simulink model "lawsdigital11"  (R2022b)
settings: Solver=VariableStepAuto  StartTime=0.0  StopTime=10.0  RelTol=1e-3
settings Model: Creator=vijit  LastModifiedBy=vijit

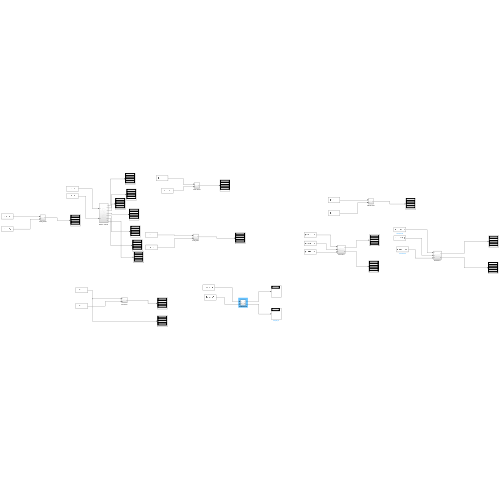
[thumbnail: Simulink's stored preview of the top-level diagram]
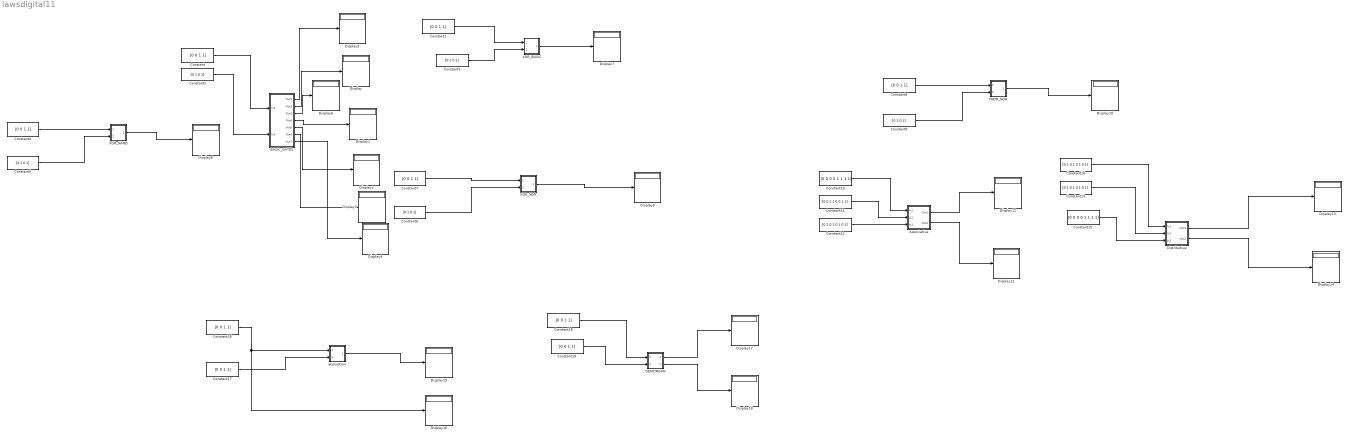
== system lawsdigital11 ==
  Associative : Subsystem
  BASIC_GATES : Subsystem
  Constant{,2,4,7..8,16..19} (9 alike) : Constant  Value=[0 0 1 1]
  Constant{1,3,5..6,9} (5 alike) : Constant  Value=[0 1 0 1]
  Constant10 : Constant  Value=[0 0 0 0 1 1 1 1]
  Constant11 : Constant  Value=[0 0 1 1 0 0 1 1]
  Constant12 : Constant  Value=[0 1 0 1 0 1 0 1]
  Constant13 : Constant  Value=[0 1 0 1 0 1 0 1]
  Constant14 : Constant  Value=[0 1 0 1 0 1 0 1]
  Constant15 : Constant  Value=[0 0 0 0 1 1 1 1]
  DEMORGAN : Subsystem
  Display{,1..18} (19 alike) : Display
  Distributive : Subsystem
  XNOR_NOR : Subsystem
  XOR_BASIC : Subsystem
  XOR_NAND : Subsystem
  XOR_NOR : Subsystem
  absorption : Subsystem
  wires:
  Constant3/1 -> XOR_BASIC/2(In2)
  Constant2/1 -> XOR_BASIC/1(In1)
  XOR_BASIC/1(Out1) -> Display7/1
  Constant/1 -> BASIC_GATES/1(In1)
  Constant1/1 -> BASIC_GATES/2(In2)
  BASIC_GATES/1(Out1) -> Display5/1
  BASIC_GATES/2(Out2) -> Display/1
  BASIC_GATES/3(Out3) -> Display6/1
  BASIC_GATES/4(Out4) -> Display1/1
  BASIC_GATES/5(Out5) -> Display2/1
  BASIC_GATES/6(Out6) -> Display3/1
  BASIC_GATES/7(Out7) -> Display4/1
  Constant4/1 -> XOR_NAND/1(In1)
  Constant5/1 -> XOR_NAND/2(In2)
  XOR_NAND/1(Out1) -> Display8/1
  Constant7/1 -> XOR_NOR/1(In1)
  Constant6/1 -> XOR_NOR/2(In2)
  XOR_NOR/1(Out1) -> Display9/1
  Constant8/1 -> XNOR_NOR/1(In1)
  Constant9/1 -> XNOR_NOR/2(In2)
  XNOR_NOR/1(Out1) -> Display10/1
  Constant10/1 -> Associative/1(In1)
  Constant11/1 -> Associative/2(In2)
  Constant12/1 -> Associative/3(In3)
  Associative/1(Out1) -> Display11/1
  Associative/2(Out2) -> Display12/1
  Constant14/1 -> Distributive/1(In1)
  Constant13/1 -> Distributive/2(In2)
  Constant15/1 -> Distributive/3(In3)
  Distributive/1(Out1) -> Display13/1
  Distributive/2(Out2) -> Display14/1
  Constant16/1 -> absorption/1(In1), Display16/1
  Constant17/1 -> absorption/2(In2)
  absorption/1(Out1) -> Display15/1
  Constant18/1 -> DEMORGAN/1(In1)
  Constant19/1 -> DEMORGAN/2(In2)
  DEMORGAN/1(Out1) -> Display17/1
  DEMORGAN/2(Out2) -> Display18/1

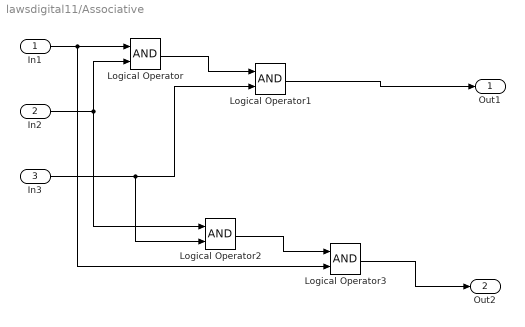
== system lawsdigital11/Associative ==
  In1 : Inport
  In2 : Inport  Port=2
  In3 : Inport  Port=3
  Logical Operator{,1..3} (4 alike) : Logic  AllPortsSameDT=off  OutDataTypeStr=boolean
  Out1 : Outport
  Out2 : Outport  Port=2
  wires:
  In3/1 -> Logical Operator2/2, Logical Operator1/2
  Logical Operator2/1 -> Logical Operator3/1
  In1/1 -> Logical Operator3/2, Logical Operator/1
  Logical Operator3/1 -> Out2/1
  In2/1 -> Logical Operator/2, Logical Operator2/1
  Logical Operator/1 -> Logical Operator1/1
  Logical Operator1/1 -> Out1/1

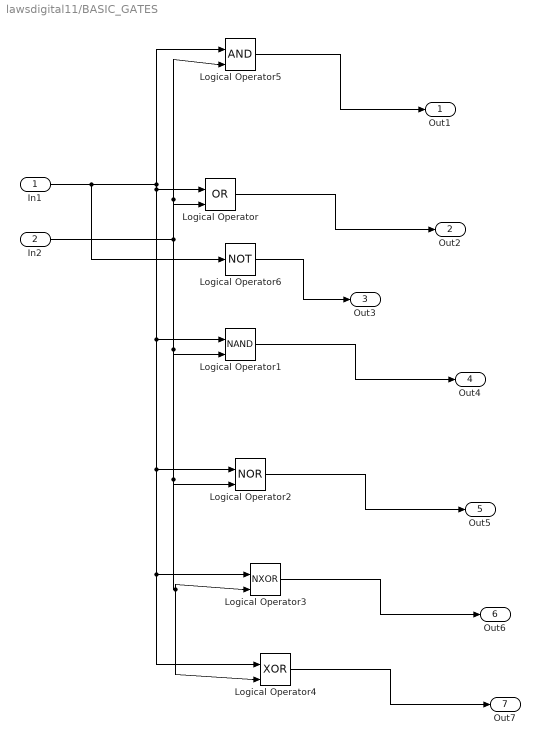
== system lawsdigital11/BASIC_GATES ==
  In1 : Inport
  In2 : Inport  Port=2
  Logical Operator : Logic  Operator=OR  IconShape=distinctive  AllPortsSameDT=off  OutDataTypeStr=boolean
  Logical Operator1 : Logic  Operator=NAND  IconShape=distinctive  AllPortsSameDT=off  OutDataTypeStr=boolean
  Logical Operator2 : Logic  Operator=NOR  IconShape=distinctive  AllPortsSameDT=off  OutDataTypeStr=boolean
  Logical Operator3 : Logic  Operator=NXOR  IconShape=distinctive  AllPortsSameDT=off  OutDataTypeStr=boolean
  Logical Operator4 : Logic  Operator=XOR  IconShape=distinctive  AllPortsSameDT=off  OutDataTypeStr=boolean
  Logical Operator5 : Logic  IconShape=distinctive  AllPortsSameDT=off  OutDataTypeStr=boolean
  Logical Operator6 : Logic  Operator=NOT  IconShape=distinctive  AllPortsSameDT=off  OutDataTypeStr=boolean
  Out1 : Outport
  Out2 : Outport  Port=2
  Out3 : Outport  Port=3
  Out4 : Outport  Port=4
  Out5 : Outport  Port=5
  Out6 : Outport  Port=6
  Out7 : Outport  Port=7
  wires:
  Logical Operator3/1 -> Out6/1
  In1/1 -> Logical Operator6/1, Logical Operator/1, Logical Operator4/1, Logical Operator3/1, Logical Operator2/1, Logical Operator1/1, Logical Operator5/1
  In2/1 -> Logical Operator5/2, Logical Operator/2, Logical Operator4/2, Logical Operator3/2, Logical Operator2/2, Logical Operator1/2
  Logical Operator1/1 -> Out4/1
  Logical Operator2/1 -> Out5/1
  Logical Operator/1 -> Out2/1
  Logical Operator4/1 -> Out7/1
  Logical Operator5/1 -> Out1/1
  Logical Operator6/1 -> Out3/1

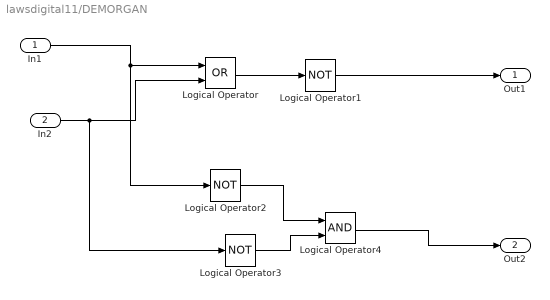
== system lawsdigital11/DEMORGAN ==
  In1 : Inport
  In2 : Inport  Port=2
  Logical Operator : Logic  Operator=OR  AllPortsSameDT=off  OutDataTypeStr=boolean
  Logical Operator1 : Logic  Operator=NOT  AllPortsSameDT=off  OutDataTypeStr=boolean
  Logical Operator2 : Logic  Operator=NOT  AllPortsSameDT=off  OutDataTypeStr=boolean
  Logical Operator3 : Logic  Operator=NOT  AllPortsSameDT=off  OutDataTypeStr=boolean
  Logical Operator4 : Logic  AllPortsSameDT=off  OutDataTypeStr=boolean
  Out1 : Outport
  Out2 : Outport  Port=2
  wires:
  Logical Operator1/1 -> Out1/1
  In1/1 -> Logical Operator2/1, Logical Operator/1
  Logical Operator4/1 -> Out2/1
  Logical Operator/1 -> Logical Operator1/1
  Logical Operator2/1 -> Logical Operator4/1
  In2/1 -> Logical Operator3/1, Logical Operator/2
  Logical Operator3/1 -> Logical Operator4/2

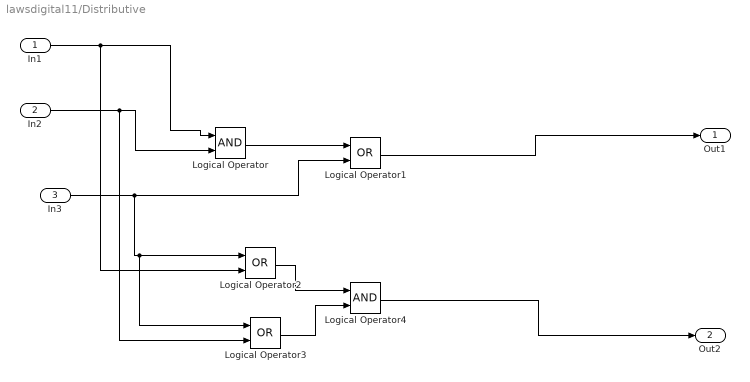
== system lawsdigital11/Distributive ==
  In1 : Inport
  In2 : Inport  Port=2
  In3 : Inport  Port=3
  Logical Operator : Logic  AllPortsSameDT=off  OutDataTypeStr=boolean
  Logical Operator1 : Logic  Operator=OR  AllPortsSameDT=off  OutDataTypeStr=boolean
  Logical Operator2 : Logic  Operator=OR  AllPortsSameDT=off  OutDataTypeStr=boolean
  Logical Operator3 : Logic  Operator=OR  AllPortsSameDT=off  OutDataTypeStr=boolean
  Logical Operator4 : Logic  AllPortsSameDT=off  OutDataTypeStr=boolean
  Out1 : Outport
  Out2 : Outport  Port=2
  wires:
  Logical Operator3/1 -> Logical Operator4/2
  Logical Operator/1 -> Logical Operator1/1
  In1/1 -> Logical Operator2/2, Logical Operator/1
  In3/1 -> Logical Operator3/1, Logical Operator2/1, Logical Operator1/2
  Logical Operator2/1 -> Logical Operator4/1
  Logical Operator4/1 -> Out2/1
  In2/1 -> Logical Operator3/2, Logical Operator/2
  Logical Operator1/1 -> Out1/1

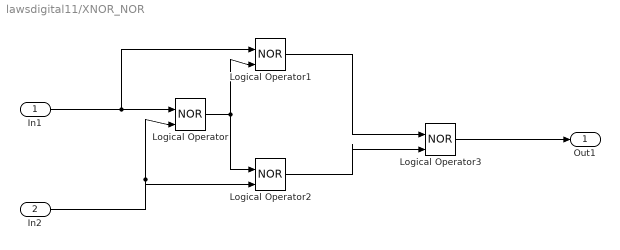
== system lawsdigital11/XNOR_NOR ==
  In1 : Inport
  In2 : Inport  Port=2
  Logical Operator{,1..3} (4 alike) : Logic  Operator=NOR  IconShape=distinctive  AllPortsSameDT=off  OutDataTypeStr=boolean
  Out1 : Outport
  wires:
  Logical Operator2/1 -> Logical Operator3/2
  In1/1 -> Logical Operator1/1, Logical Operator/1
  Logical Operator/1 -> Logical Operator1/2, Logical Operator2/1
  Logical Operator1/1 -> Logical Operator3/1
  In2/1 -> Logical Operator/2, Logical Operator2/2
  Logical Operator3/1 -> Out1/1

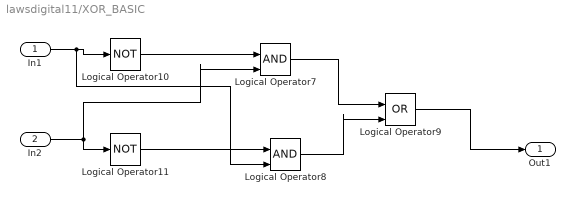
== system lawsdigital11/XOR_BASIC ==
  In1 : Inport
  In2 : Inport  Port=2
  Logical Operator10 : Logic  Operator=NOT  IconShape=distinctive  AllPortsSameDT=off  OutDataTypeStr=boolean
  Logical Operator11 : Logic  Operator=NOT  IconShape=distinctive  AllPortsSameDT=off  OutDataTypeStr=boolean
  Logical Operator7 : Logic  IconShape=distinctive  AllPortsSameDT=off  OutDataTypeStr=boolean
  Logical Operator8 : Logic  IconShape=distinctive  AllPortsSameDT=off  OutDataTypeStr=boolean
  Logical Operator9 : Logic  Operator=OR  IconShape=distinctive  AllPortsSameDT=off  OutDataTypeStr=boolean
  Out1 : Outport
  wires:
  Logical Operator8/1 -> Logical Operator9/2
  Logical Operator7/1 -> Logical Operator9/1
  In2/1 -> Logical Operator7/2, Logical Operator11/1
  Logical Operator11/1 -> Logical Operator8/1
  Logical Operator9/1 -> Out1/1
  In1/1 -> Logical Operator8/2, Logical Operator10/1
  Logical Operator10/1 -> Logical Operator7/1

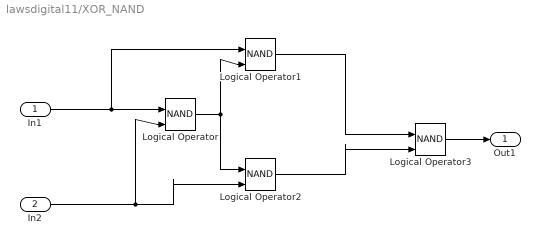
== system lawsdigital11/XOR_NAND ==
  In1 : Inport
  In2 : Inport  Port=2
  Logical Operator{,1..3} (4 alike) : Logic  Operator=NAND  IconShape=distinctive  AllPortsSameDT=off  OutDataTypeStr=boolean
  Out1 : Outport
  wires:
  In2/1 -> Logical Operator/2, Logical Operator2/2
  Logical Operator/1 -> Logical Operator1/2, Logical Operator2/1
  Logical Operator3/1 -> Out1/1
  In1/1 -> Logical Operator1/1, Logical Operator/1
  Logical Operator1/1 -> Logical Operator3/1
  Logical Operator2/1 -> Logical Operator3/2

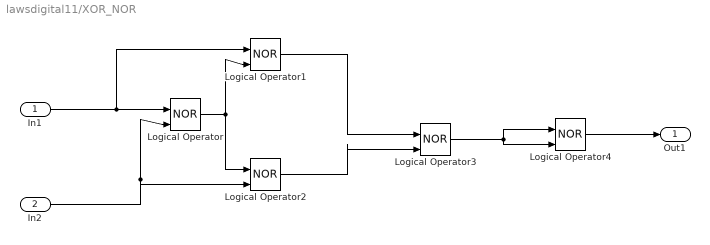
== system lawsdigital11/XOR_NOR ==
  In1 : Inport
  In2 : Inport  Port=2
  Logical Operator{,1..4} (5 alike) : Logic  Operator=NOR  IconShape=distinctive  AllPortsSameDT=off  OutDataTypeStr=boolean
  Out1 : Outport
  wires:
  Logical Operator3/1 -> Logical Operator4/2, Logical Operator4/1
  In2/1 -> Logical Operator/2, Logical Operator2/2
  Logical Operator4/1 -> Out1/1
  Logical Operator/1 -> Logical Operator1/2, Logical Operator2/1
  In1/1 -> Logical Operator1/1, Logical Operator/1
  Logical Operator2/1 -> Logical Operator3/2
  Logical Operator1/1 -> Logical Operator3/1

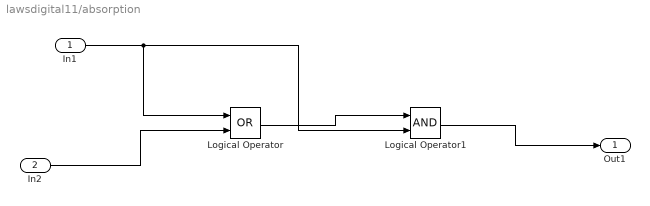
== system lawsdigital11/absorption ==
  In1 : Inport
  In2 : Inport  Port=2
  Logical Operator : Logic  Operator=OR  AllPortsSameDT=off  OutDataTypeStr=boolean
  Logical Operator1 : Logic  AllPortsSameDT=off  OutDataTypeStr=boolean
  Out1 : Outport
  wires:
  Logical Operator1/1 -> Out1/1
  In1/1 -> Logical Operator1/2, Logical Operator/1
  Logical Operator/1 -> Logical Operator1/1
  In2/1 -> Logical Operator/2
